simulink model "RSP"  (R2023a)
settings: Solver=FixedStepDiscrete  StartTime=0.0  StopTime=1.1*pri*N_observation  FixedStep=1.220703125E-8  RelTol=1e-3  EnableMultiTasking=on
model workspace (MAT data in the model file):
  Lambda : Simulink.Parameter (value not decoded)
  N_observation : Simulink.Parameter (value not decoded)
  N_sample : Simulink.Parameter (value not decoded)
  T_sampling : Simulink.Parameter (value not decoded)
  T_symbol : Simulink.Parameter (value not decoded)
  pri : Simulink.Parameter (value not decoded)
  symbol_delay : Simulink.Parameter (value not decoded)
symbols that are objects in the model workspace (value not decoded): Lambda, N_observation, N_sample, symbol_delay, T_sampling
libraries: hdlsllib x4, dsphdlxfrm2 x1
(part 37 of 49)

== matlab function RSP/Range Processor/Range Calculator/Correlator ==
  settings: fimath=fimath('OverflowAction','Saturate','RoundingMethod','Zero','ProductMode','KeepMSB')
  data: max_corr_lag output; x input; y input; obs_sample output; counter input
function [max_corr_lag, obs_sample]  = fcn(x,y,counter)
%#codegen

N = uint16(length(x));
% out = fi(zeros(1,out_len),1,64,0);
idx = uint16(0);
max = fi(1,1,128);

if counter >= 16383 
    for m = (1:N)
        sum = fi(1,1,128);
        % len_xcorr = out_len-m;
        
        for n = 1:N
            if n <= N-m
                sum = accumpos(sum, y(n+m-1) * x(n), 'Convergent', 'Saturate');
            end
        end
        
        % out(m) = sum;
    
        if(sum > max) 
            max = sum; 
            idx = m;
        end
    end

    % max_corr = max;
    
    if(idx == 0)
        max_corr_lag = uint16(0);
    else
        max_corr_lag = uint16(idx);
    end
    
    obs_sample = y(max_corr_lag+3);
else
    max_corr_lag = uint16(0);
    obs_sample = y(max_corr_lag+3);
end
